simulink model "cv_7_sim"  (R2019b)
settings: Solver=FixedStepAuto  StartTime=0.0  StopTime=Tsim  FixedStep=Ts  RelTol=1e-3
values from neighbouring files (symbols this model uses):
  beta = 2.0*sqrt(g/l)    [cv_7.m]
  g = 9.81    [cv_7.m]
  l = 1    [cv_7.m]
  m = 1    [cv_7.m]
  omega_0 = 0    [cv_7.m]
  phi_0 = y_pb_prevod*0.0    [cv_7.m]
  T_step = Tsim/2    (= 7.5)    [cv_7.m]
  Ts = 0.1    [cv_7.m]
  u_pb = m*g*l*sin(y_pb_prevod)    [cv_7.m]
  u_pb_h = m*g*l*sin(y_pb_h_prevod)    [cv_7.m]
undefined symbols (not defined in the file or in its folder): u_0
libraries: simulink x1
settings Model: Creator=Martin Dodek  LastModifiedBy=Martin Dodek

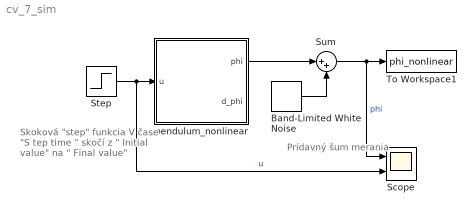
== system cv_7_sim ==
  note: Prídavný šum merania
  note: Skoková "step" funkcia
      | V čase "S tep time "
      | skočí z " Initial value" na " Final value"
  Band-Limited White Noise : simulink/Sources/Band-Limited White Noise  Cov=1e-6  Ts=Ts  seed=[23341]
  Scope : Scope  NumInputPorts=2
  Step : Step  Time=T_step  Before=u_pb  After=u_pb_h  SampleTime=0
  Sum : Sum  Inputs=|++
  To Workspace1 : ToWorkspace  VariableName=phi_nonlinear  SampleTime=-1
  pendulum_nonlinear : Subsystem
  wires:
  Step/1 -> Scope/2, pendulum_nonlinear/1(u)  "u"
  pendulum_nonlinear/1(phi) -> Sum/1
  Band-Limited White Noise/1 -> Sum/2
  Sum/1 -> Scope/1, To Workspace1/1  "phi"

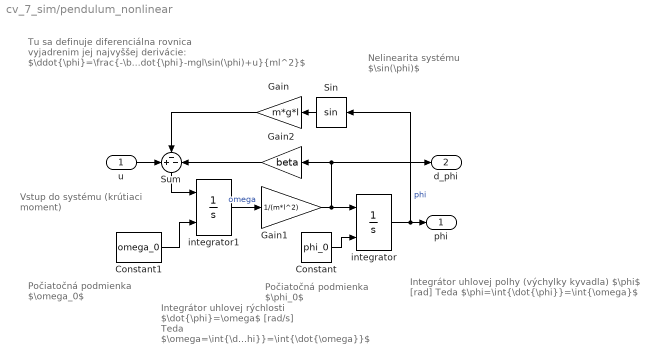
== system cv_7_sim/pendulum_nonlinear ==
  note: Počiatočná podmienka
      | $\phi_0$
  note: Počiatočná podmienka
      | $\omega_0$
  note: Integrátor uhlovej polhy (výchylky kyvadla) $\phi$ [rad]
      | Teda $\phi=\int{\dot{\phi}}=\int{\omega}$
  note: Nelinearita systému
      | $\sin(\phi)$
  note: Tu sa definuje diferenciálna rovnica vyjadrenim jej najvyššej derivácie:
      | $\ddot{\phi}=\frac{-\beta\dot{\phi}-mgl\sin(\phi)+u}{ml^2}$
  note: Vstup do systému (krútiaci moment)
  note: Integrátor uhlovej rýchlosti $\dot{\phi}=\omega$ [rad/s]
      | Teda $\omega=\int{\ddot{\phi}}=\int{\dot{\omega}}$
  u : Inport
  Constant : Constant  Value=phi_0
  Constant1 : Constant  Value=omega_0
  Gain : Gain  Gain=m*g*l
  Gain1 : Gain  Gain=1/(m*l^2)
  Gain2 : Gain  Gain=beta
  Sin : Trigonometry
  Sum : Sum  Inputs=+--
  integrator : Integrator  InitialConditionSource=external  InitialCondition=u_0
  integrator1 : Integrator  InitialConditionSource=external  InitialCondition=u_0
  phi : Outport
  d_phi : Outport  Port=2
  wires:
  integrator/1 -> Sin/1, phi/1  "phi"
  Constant1/1 -> integrator1/2
  integrator1/1 -> Gain1/1  "omega"
  Constant/1 -> integrator/2
  Sin/1 -> Gain/1
  Gain1/1 -> d_phi/1, Gain2/1, integrator/1
  Sum/1 -> integrator1/1
  u/1 -> Sum/1
  Gain2/1 -> Sum/3
  Gain/1 -> Sum/2
